simulink model "simu_21uec072"  (R2022b)
settings: Solver=VariableStepAuto  StartTime=0.0  StopTime=0  RelTol=1e-3
settings Model: Creator=DSP-27  LastModifiedBy=DSP-27

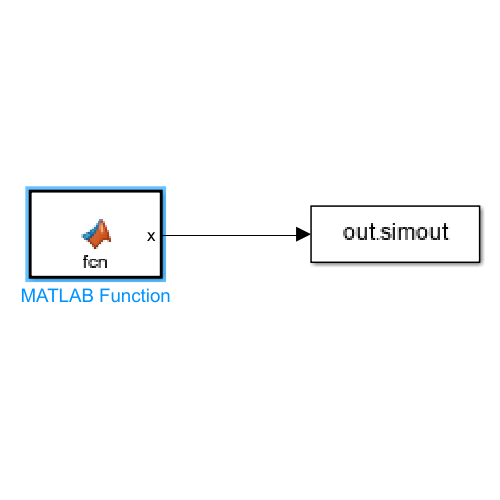
[thumbnail: Simulink's stored preview of the top-level diagram]
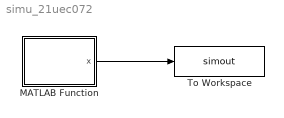
== system simu_21uec072 ==
  MATLAB Function : MATLAB Function  TreatAsAtomicUnit=on
  To Workspace : ToWorkspace  VariableName=simout  SampleTime=-1
      settings: Save2DSignal=2-D array (concatenate along first dimension)
  wires:
  MATLAB Function/1(x) -> To Workspace/1

== matlab function simu_21uec072/MATLAB Function ==
  data: x output
function x = fcn()
x=[1,2,3,4];
z=complex(zeros(1,length(x)));
W = exp(-1i*pi/2);
k11 = x(1) + x(3);
k12 = x(1) - x(3);
k21 = x(2) + x(4);
k22 = x(2) - x(4);

z(1) = k11 + k21;
z(2) = k12 + k22*W;
z(3) = k11 - k21;
z(4) = k12 - k22*W;
end
